simulink model "sf_hierarchy"  (R2015b)
settings: Solver=FixedStepDiscrete  SolverMode=SingleTasking  StartTime=0.0  StopTime=1/10  RelTol=1e-3
settings Model: Creator=at-mt  LastModifiedBy=amatsumo
settings DataIOCC: SaveFormat=Array  SignalLoggingSaveFormat=ModelDataLogs  SaveOutput=off  SignalLogging=off  SaveTime=off
settings OptimizationCC: BlockReduction=off  ConditionallyExecuteInputs=off  DefaultParameterBehavior=Inlined  ExpressionDepthLimit=2147483647
settings DebuggingCC: AlgebraicLoopMsg=error  UnderspecifiedInitializationDetection=Classic  MergeDetectMultiDrivingBlocksExec=none  SolverPrmCheckMsg=warning  SingleTaskRateTransMsg=error  FcnCallInpInsideContextMsg=UseLocalSettings  StateNameClashWarn=warning
settings HardwareCC: ProdBitPerPointer=32  ProdLargestAtomicFloat=None  ProdIntDivRoundTo=Undefined  ProdEndianess=Unspecified  ProdWordSize=32  ProdHWDeviceType=ASIC/FPGA->ASIC/FPGA  ProdEqTarget=off
settings SFSimCC: SimParseCustomCode=off
settings GRTTargetCC: GeneratePreprocessorConditionals=Disable all  CombineOutputUpdateFcns=off  GRTInterface=on
settings ConfigComp: CovMetricSettings=dcmw  CovSFcnEnable=off

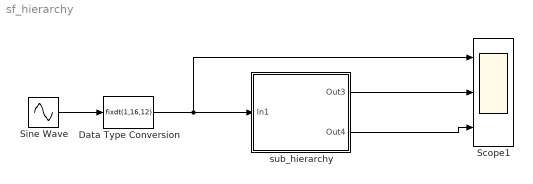
== system sf_hierarchy ==
  Data Type Conversion : DataTypeConversion  OutDataTypeStr=fixdt(1,16,12)
  Scope1 : Scope  NumInputPorts=3
  Sine Wave : Sin  Amplitude=4  Bias=0.2  Frequency=2*pi*20  SampleTime=1/100
  sub_hierarchy : Subsystem
  wires:
  Sine Wave/1 -> Data Type Conversion/1
  Data Type Conversion/1 -> Scope1/1, sub_hierarchy/1(In1)
  sub_hierarchy/1(Out3) -> Scope1/2
  sub_hierarchy/2(Out4) -> Scope1/3

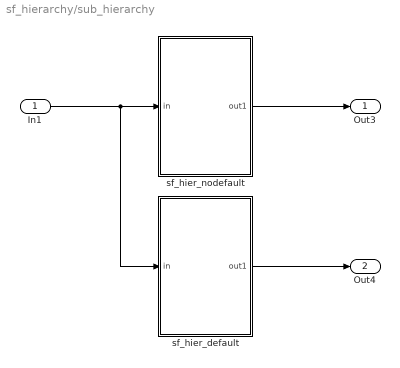
== system sf_hierarchy/sub_hierarchy ==
  In1 : Inport
  sf_hier_default : Stateflow chart  TreatAsAtomicUnit=on
  sf_hier_nodefault : Stateflow chart  TreatAsAtomicUnit=on
  Out3 : Outport
  Out4 : Outport  Port=2
  wires:
  In1/1 -> sf_hier_nodefault/1(in), sf_hier_default/1(in)
  sf_hier_default/1(out1) -> Out4/1
  sf_hier_nodefault/1(out1) -> Out3/1

== stateflow chart sf_hierarchy/sub_hierarchy/sf_hier_default ==
  settings: updateMethod=DISCRETE  stateMachineType=MOORE_MACHINE  executeAtInitialization=1  initializeOutput=1
  state Init/
    out1 = 2;
  state On_Parent
    state On1/
      out1 = 1;
    state On2/
      out1 = 0;
    (default) -> On1
    On2 -> On1
    On1 -> On2 [order 2]
  Init -> Init [order 2]
  (default) -> Init
  Init -> On1 [order 1] : [in < 0]
  On1 -> Init [order 1] : [in >= 0]
  data: in input fixdt(1,16,12) size=1; out1 output int16

== stateflow chart sf_hierarchy/sub_hierarchy/sf_hier_nodefault ==
  settings: updateMethod=DISCRETE  stateMachineType=MOORE_MACHINE  executeAtInitialization=1  initializeOutput=1
  state Init/
    out1 = 2;
  state On_Parent
    state On1/
      out1 = 1;
    state On2/
      out1 = 0;
    On2 -> On1
    On1 -> On2 [order 1]
  Init -> Init [order 2]
  (default) -> Init
  Init -> On1 [order 1] : [in < 0]
  On1 -> Init [order 2] : [in >= 0]
  data: in input fixdt(1,16,12) size=1; out1 output int16
